simulink model "identification"  (R2020a)
settings: Solver=FixedStepDiscrete  StartTime=0.0  StopTime=inf  FixedStep=Te  RelTol=1e-3
values from neighbouring files (symbols this model uses):
  Te = 0.01    [identificat.m]    (also in projet.mat)
undefined symbols (not defined in the file or in its folder): National_Instruments, PCI
libraries: sldrtlib x2, simulink x1
settings Model: Creator=soual  LastModifiedBy=soual
settings RTWCC: Description=Simulink Desktop Real-Time  SystemTargetFile=sldrt.tlc  TemplateMakefile=sldrt.tmf  RTWCompilerOptimization=on
settings CodeAppCC: MaxIdLength=95
settings SimulinkDesktopRealTimeCC: TargetPreCompLibLocation=C:\Program Files\MATLAB\R2020a\toolbox\sldrt\lib\win64

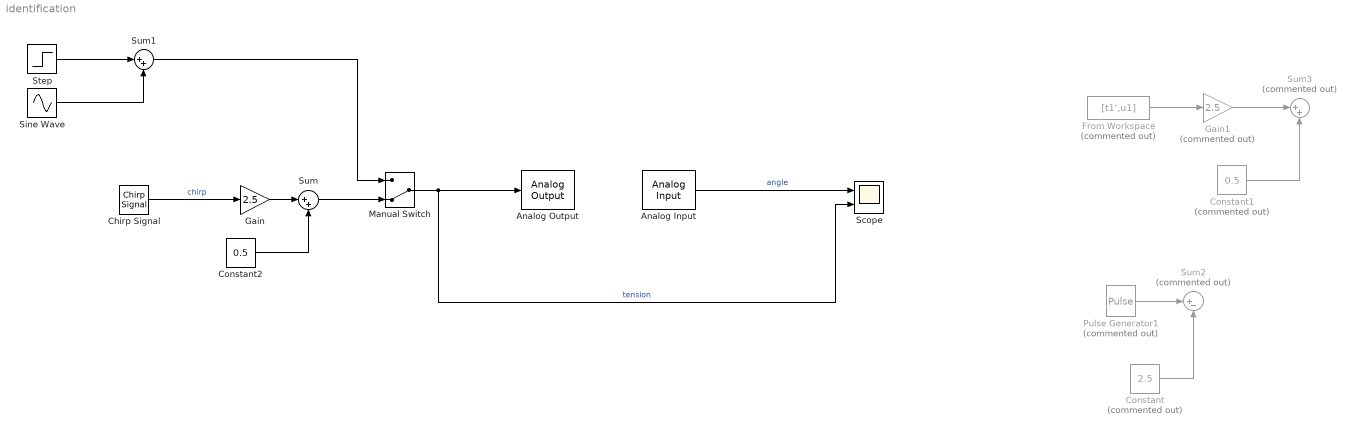
== system identification ==
  Analog Input : sldrtlib/Analog Input  SampleTime=Te  MaxMissedTicks=10  ShowMissedTicks=off  YieldWhenWaiting=off  DrvName=National_Instruments/PCI-6024E  DrvAddress=4294967295  DrvOptions=[0 0 0 0 0 0]  Channels=1  RangeMode=1  VoltRange=1  DataType=1
      settings: AttributesFormatString=National Instruments\nPCI-6024E [auto]
  Analog Output : sldrtlib/Analog Output  SampleTime=Te  MaxMissedTicks=10  ShowMissedTicks=off  YieldWhenWaiting=off  DrvName=National_Instruments/PCI-6024E  DrvAddress=4294967295  DrvOptions=[0 0 0 0 0 0]  Channels=1  RangeMode=1  VoltRange=1  InitialValue=0  FinalValue=0
      settings: AttributesFormatString=National Instruments\nPCI-6024E [auto]
  Chirp Signal : simulink/Sources/Chirp Signal  f1=0.3  T=60  f2=5
  Constant : Constant  Commented=on  Value=2.5
  Constant1 : Constant  Commented=on  Value=0.5
  Constant2 : Constant  Value=0.5
  From Workspace : FromWorkspace  Commented=on  VariableName=[t1',u1]  SampleTime=Te
  Gain : Gain  Gain=2.5
  Gain1 : Gain  Commented=on  Gain=2.5
  Manual Switch : ManualSwitch  CurrentSetting=0
  Pulse Generator1 : DiscretePulseGenerator  Commented=on  PulseType=Time based  Amplitude=6  Period=4  PulseWidth=50
  Scope : Scope  NumInputPorts=2
  Sine Wave : Sin  Amplitude=2  Frequency=0.5  SampleTime=Te
  Step : Step  Before=5  After=-1  SampleTime=Te
  Sum : Sum  Inputs=|++
  Sum1 : Sum  Inputs=|++
  Sum2 : Sum  Commented=on  Inputs=|+-
  Sum3 : Sum  Commented=on  Inputs=|++
  wires:
  Analog Input/1 -> Scope/1  "angle"
  Manual Switch/1 -> Scope/2, Analog Output/1  "tension"
  Chirp Signal/1 -> Gain/1  "chirp"
  Gain/1 -> Sum/1
  Constant2/1 -> Sum/2
  Sine Wave/1 -> Sum1/2
  Step/1 -> Sum1/1
  Sum1/1 -> Manual Switch/1
  From Workspace/1 -> Gain1/1
  Pulse Generator1/1 -> Sum2/1
  Constant/1 -> Sum2/2
  Gain1/1 -> Sum3/1
  Constant1/1 -> Sum3/2
  Sum/1 -> Manual Switch/2
